simulink model "sim_sistema_1"  (Simulink 7.5)
settings: Solver=ode3  StartTime=0.0  StopTime=5  FixedStep=1e-4  RelTol=1e-3
values from neighbouring files (symbols this model uses):
  C = zpk(w2,w1,a)    [network_delay.m]    (also in network_foward.m = zpk(-w2,-w1,a))
  K = Kp*6*21    (= 0)    [network_delay.m]
undefined symbols (not defined in the file or in its folder): A, B, D
settings Model: Creator=taniel.franklin  LastModifiedBy=taniel.franklin

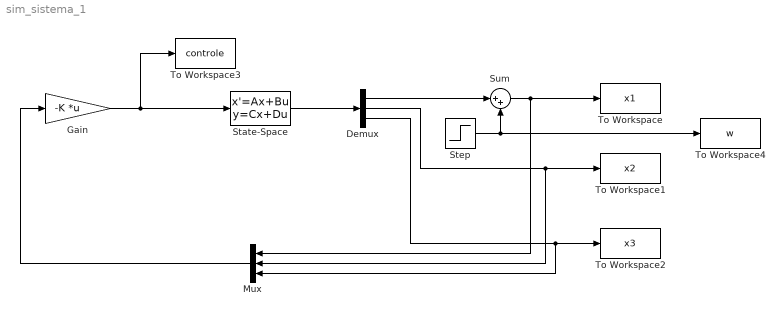
== system sim_sistema_1 ==
  Demux : Demux  Outputs=3
  Gain : Gain  Gain=-K  Multiplication=Matrix(K*u)  ParameterDataType=fixdt(1, 16)  ParameterScaling=2^0  OutDataType=fixdt(1, 16)  OutScaling=2^0
  Mux : Mux  Inputs=3
  State-Space : StateSpace  A=A  B=B  C=C  D=D  X0=[0;0;0]
  Step : Step  SampleTime=0
  Sum : Sum  Inputs=|++  OutDataType=fixdt(1, 16)  OutScaling=2^0
  To Workspace : ToWorkspace  VariableName=x1  SampleTime=-1  SaveFormat=Structure With Time
  To Workspace1 : ToWorkspace  VariableName=x2  SampleTime=-1  SaveFormat=Structure With Time
  To Workspace2 : ToWorkspace  VariableName=x3  SampleTime=-1  SaveFormat=Structure With Time
  To Workspace3 : ToWorkspace  VariableName=controle  SampleTime=-1  SaveFormat=Structure With Time
  To Workspace4 : ToWorkspace  VariableName=w  SampleTime=-1  SaveFormat=Structure With Time
  wires:
  State-Space/1 -> Demux/1
  Demux/2 -> To Workspace1/1, Mux/2
  Demux/3 -> To Workspace2/1, Mux/3
  Gain/1 -> State-Space/1, To Workspace3/1
  Sum/1 -> To Workspace/1, Mux/1
  Demux/1 -> Sum/1
  Step/1 -> Sum/2, To Workspace4/1
  Mux/1 -> Gain/1
